simulink model "modeling_aa"  (R2024a)
settings: Solver=VariableStepAuto  StartTime=0.0  StopTime=25  FixedStep=0.000001  AbsTol=1e-4
values from neighbouring files (symbols this model uses):
  A = [0, 1; 9, 2]    [main.m]    (also in prep.m = [0 1; 9 2])
  A0f = [0 1 0 0 ... (first row only)    [prep.m]
  b = [9; 5]    [main.m]    (also in prep.m)
  C = [3, 3]    [main.m]    (also in prep.m = [3 3])
  d = b    [main.m]    (also in prep.m = [9; 5])
  N = b0f/d    [prep.m]
  P = lyap(Acl', Q_lyap)    [main.m]    (also in prep.m = lyap(Am', Q))
undefined symbols (not defined in the file or in its folder): K
settings Model: Creator=ventus  LastModifiedBy=ventus
settings OptimizationCC: EnhancedBackFolding=on  PassReuseOutputArgsAs=Individual arguments  ZeroExternalMemoryAtStartup=off  ZeroInternalMemoryAtStartup=off  MaxStackSize=64  OptimizeBlockOrder=speed  DifferentSizesBufferReuse=on  OptimizationCustomize=off  EfficientTunableParamExpr=on
settings DebuggingCC: ParameterTunabilityLossMsg=error
settings SFSimCC: MATLABDynamicMemAlloc=off
settings RTWCC: Description=Embedded Coder  SystemTargetFile=ert.tlc  HardwareBoard=Robot Operating System 2 (ROS 2)  TLCOptions="-aInlineSetEventsForThisBaseRateFcn=TLC_FALSE -aSuppressMultiTaskScheduler=TLC_FALSE  -aRateBasedStepFcn=0"  TemplateMakefile=ert_default_tmf  Toolchain=Colcon Tools  TargetLang=C++
settings CodeAppCC: ForceParamTrailComments=on  IgnoreCustomStorageClasses=off  OperatorAnnotations=on  SimulinkDataObjDesc=on  SFDataObjDesc=on  InsertBlockDesc=on
settings ERTTargetCC: CodeInterfacePackaging=C++ class  RootIOFormat=Structure reference

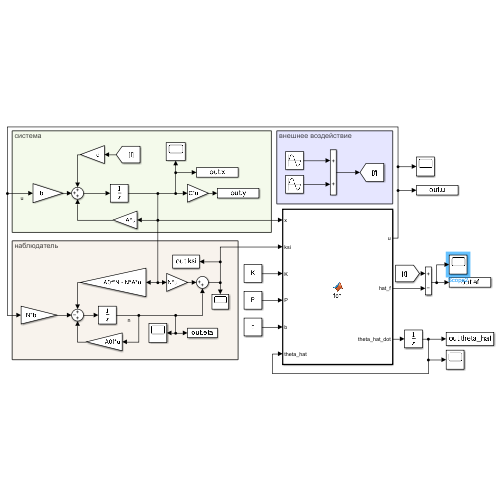
[thumbnail: Simulink's stored preview of the top-level diagram]
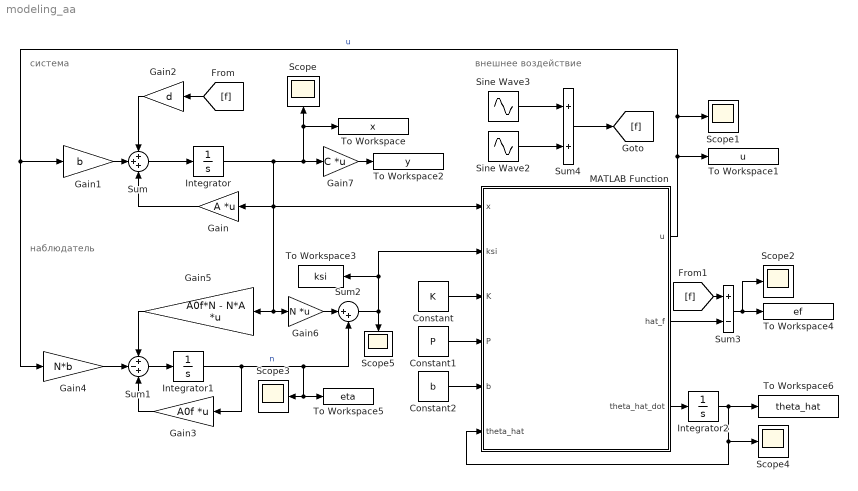
== system modeling_aa ==
  note: система
  note: наблюдатель
  note: внешнее воздействие
  Constant : Constant  Value=K  VectorParams1D=off
  Constant1 : Constant  Value=P  VectorParams1D=off
  Constant2 : Constant  Value=b  VectorParams1D=off
  Gain : Gain  Gain=A  Multiplication=Matrix(K*u)
  Gain1 : Gain  Gain=b
  Gain2 : Gain  Gain=d
  Gain3 : Gain  Gain=A0f  Multiplication=Matrix(K*u)
  Gain4 : Gain  Gain=N*b
  Gain5 : Gain  Gain=A0f*N - N*A  Multiplication=Matrix(K*u)
  Gain6 : Gain  Gain=N  Multiplication=Matrix(K*u)
  Gain7 : Gain  Gain=C  Multiplication=Matrix(K*u)
  Integrator : Integrator
  Integrator1 : Integrator
  Integrator2 : Integrator
  MATLAB Function : MATLAB Function  TreatAsAtomicUnit=on
  Scope{,1..5} (6 alike) : Scope
  Sine Wave2 : Sin  Amplitude=1/2  Frequency=9  Phase=2  SampleTime=0
  Sine Wave3 : Sin  Amplitude=1/2  Frequency=7  Phase=-16  SampleTime=0
  Sum : Sum  Inputs=+++
  Sum1 : Sum  Inputs=+-+
  Sum2 : Sum  Inputs=|++
  Sum3 : Sum  Inputs=+-
  Sum4 : Sum
  To Workspace : ToWorkspace  VariableName=x  SaveFormat=Timeseries  SampleTime=-1
  To Workspace1 : ToWorkspace  VariableName=u  SaveFormat=Timeseries  SampleTime=-1
  To Workspace2 : ToWorkspace  VariableName=y  SaveFormat=Timeseries  SampleTime=-1
  To Workspace3 : ToWorkspace  VariableName=ksi  SaveFormat=Timeseries  SampleTime=-1
  To Workspace4 : ToWorkspace  VariableName=ef  SaveFormat=Timeseries  SampleTime=-1
  To Workspace5 : ToWorkspace  VariableName=eta  SaveFormat=Timeseries  SampleTime=-1
  To Workspace6 : ToWorkspace  VariableName=theta_hat  SaveFormat=Timeseries  SampleTime=-1
  wires:
  Sum/1 -> Integrator/1
  Integrator/1 -> Gain7/1, To Workspace/1, Scope/1, MATLAB Function/1(x), Gain/1, Gain5/1, Gain6/1
  Gain/1 -> Sum/3
  Gain2/1 -> Sum/1
  Sum1/1 -> Integrator1/1
  Integrator1/1 -> Gain3/1, Sum2/2, To Workspace5/1, Scope3/1  "n"
  Gain3/1 -> Sum1/3
  Gain4/1 -> Sum1/2
  Gain5/1 -> Sum1/1
  Gain6/1 -> Sum2/1
  Sum2/1 -> MATLAB Function/2(ksi), To Workspace3/1, Scope5/1
  MATLAB Function/3(theta_hat_dot) -> Integrator2/1
  Integrator2/1 -> To Workspace6/1, MATLAB Function/6(theta_hat), Scope4/1
  MATLAB Function/1(u) -> Gain1/1, Gain4/1, Scope1/1, To Workspace1/1  "u"
  Constant/1 -> MATLAB Function/3(K)
  Constant1/1 -> MATLAB Function/4(P)
  Constant2/1 -> MATLAB Function/5(b)
  Gain1/1 -> Sum/2
  Gain7/1 -> To Workspace2/1
  Sine Wave3/1 -> Sum4/1
  Sine Wave2/1 -> Sum4/2
  [f] -> Gain2/1
  Sum4/1 -> [f]
  MATLAB Function/2(hat_f) -> Sum3/2
  [f] -> Sum3/1
  Sum3/1 -> Scope2/1, To Workspace4/1

== matlab function modeling_aa/MATLAB Function ==
  data: u output; hat_f output; x input; ksi input; K input; P input; b input; theta_hat input; theta_hat_dot output
function [u, hat_f, theta_hat_dot] = fcn(x, ksi, K, P, b, theta_hat)
gamma = 300000;
hat_f = theta_hat'*ksi;
u = -K*x -hat_f;

theta_hat_dot = gamma*ksi*b'*P*x;
